simulink model "rtwdemo_sffor"  (Simulink 7.6)
settings: Solver=FixedStepDiscrete  StartTime=0.0  StopTime=10  FixedStep=1  RelTol=1e-3  SampleTimeConstraint=STIndependent
PostLoadFcn:
  | clear;
  | rtwdemo_sffor_data
undefined symbols (not defined in the file or in its folder): P1, P2
libraries: rtwdemowidgets x2
Description:
  | Efficient Loops in Stateflow(R)
settings Model: Creator=The MathWorks Inc.  ExtModeAutoUpdateStatusClock=off
settings DataIOCC: SaveOutput=off  SaveTime=off  SignalLoggingName=logsOut
settings OptimizationCC: InlineParams=on  InlineInvariantSignals=on  StateBitsets=on  DataBitsets=on  UseTempVars=on  EfficientFloat2IntCast=on  EfficientMapNaN2IntZero=off
settings DebuggingCC: CheckExecutionContextPreStartOutputMsg=on  CheckExecutionContextRuntimeOutputMsg=on  SolverPrmCheckMsg=none  StrictBusMsg=ErrorOnBusTreatedAsVector
settings HardwareCC: ProdIntDivRoundTo=Zero  ProdEndianess=LittleEndian  ProdHWDeviceType=Generic->32-bit Embedded Processor  TargetHWDeviceType=Generic->32-bit Embedded Processor
settings ModelReferenceCC: UpdateModelReferenceTargets=IfOutOfDate
settings SFSimCC: SimParseCustomCode=off
settings RTWCC: TLCOptions=-p0 -aWarnNonSaturatedBlocks=0  Description=RTW Embedded Coder (auto configures for optimized floating-point code)  GenerateReport=on  RTWVerbose=off  ProcessScript=grt_make_rtw_hook  LaunchReport=on
settings CodeAppCC: ForceParamTrailComments=on
settings GRTTargetCC: TargetFcnLib=ansi_tfl_tmw.mat

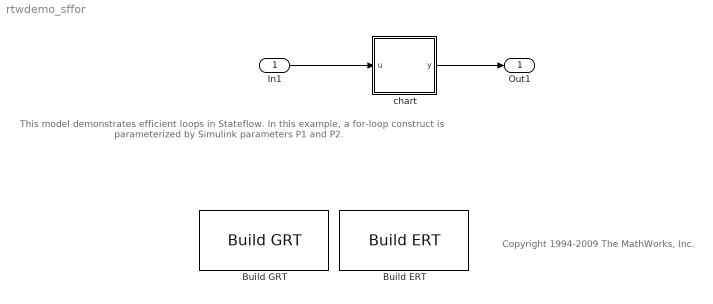
== system rtwdemo_sffor ==
  note: This model demonstrates efficient loops in Stateflow.  In this
      | example, a for-loop construct is parameterized by Simulink
      | parameters P1 and P2.
  note: Copyright 1994-2009 The MathWorks, Inc.
  In1 : Inport  OutDataTypeStr=single  PortDimensions=1
  Build ERT : rtwdemowidgets/Build ERT  SystemSampleTime=-1  attrib_overrides={}
  Build GRT : rtwdemowidgets/Build GRT  SystemSampleTime=-1  attrib_overrides={}
  chart : Stateflow chart  TreatAsAtomicUnit=on
  Out1 : Outport
  wires:
  chart/1(y) -> Out1/1
  In1/1 -> chart/1(u)

== stateflow chart chart ==
  state f [function]
    (default) -> (junction 4) : {y=0;i=P1;}
    (junction 4) -> (junction 4) [order 1] : [i<P2]{x=i;i++;}
    (junction 4) -> (junction 5) [order 2] : {y=u*x;}
  (default) -> (junction 6) : {f();}
  data: x temporary type(u) size=1; i local int8 size=1; P1 parameter double size=1; P2 parameter double size=1; y output type(u) size=1; u input double
